simulink model "sampleModel1837"  (R2023a)
settings: Solver=VariableStepAuto  StartTime=0.0  StopTime=10.0  RelTol=1e-3
libraries: simulink x3, hdlsllib x2
settings Model: Creator=user1  LastModifiedBy=user1

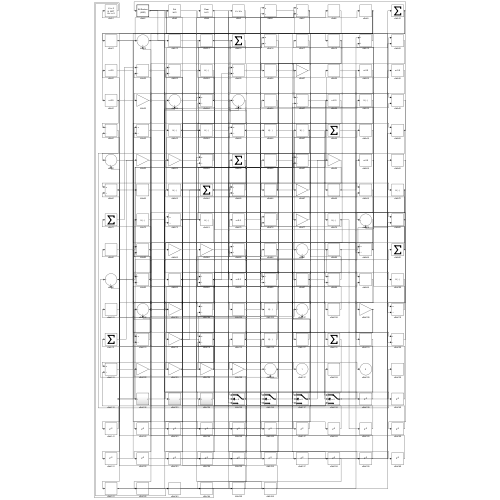
[thumbnail: Simulink's stored preview of the top-level diagram]
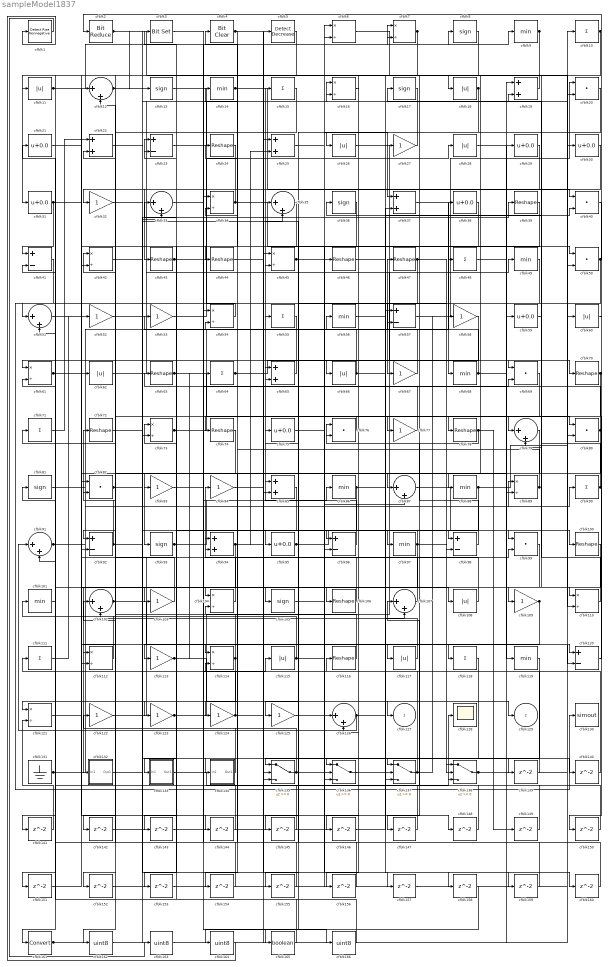
== system sampleModel1837 ==
  cfblk1 : hdlsllib/Logic and Bit Operations/Detect Rise Nonnegative  vinit=0  OutDataTypeStr=boolean
  cfblk{10,15,48,55,64,71,90,111,118} (9 alike) : Sum  Inputs=+
  cfblk{24,39,43..44,46..47,63,70,72,74,78,100,106,116} (14 alike) : Reshape
  cfblk{9,14,49,56,68,86,88,97,101,119} (10 alike) : MinMax
  cfblk{12,33,35,51,79,87,91,102,107,126} (10 alike) : Sum  Inputs=|++
  cfblk{27,32,52..53,58,67,77,83..84,103,109,113,122..125} (16 alike) : Gain
  cfblk{6..7,16,34,42,45,54,61,73,89,104,110,112,114,121} (15 alike) : Product  Inputs=*/  RndMeth=Zero  SaturateOnIntegerOverflow=on
  cfblk{8,13,17,36,81,93,105} (7 alike) : Signum
  cfblk{11,18,26,28,60,62,66,108,115,117} (10 alike) : Abs  SaturateOnIntegerOverflow=off
  cfblk{23,41,57,92,96,98,120} (7 alike) : Sum  Inputs=+-
  cfblk128 : Scope
  cfblk130 : ToWorkspace  VariableName=simout  SaveFormat=Timeseries  SampleTime=-1
  cfblk131 : Ground
  cfblk132 : Subsystem
      settings: LibrarySourceBlock=|
      | hdlsllib/Ports &
      | Subsystems/Subsystem
  cfblk133 : Subsystem
      settings: LibrarySourceBlock=|
      | hdlsllib/Ports &
      | Subsystems/Subsystem
  cfblk134 : Subsystem
      settings: LibrarySourceBlock=|
      | hdlsllib/Ports &
      | Subsystems/Subsystem
  cfblk{135..138} (4 alike) : Switch  SaturateOnIntegerOverflow=off  InputSameDT=off
  cfblk{139..160} (22 alike) : Delay  SampleTime=1
  cfblk161 : DataTypeConversion  SaturateOnIntegerOverflow=off  RndMeth=Floor
  cfblk{162..164,166} (4 alike) : DataTypeConversion  OutDataTypeStr=uint8  SaturateOnIntegerOverflow=off  RndMeth=Floor
  cfblk165 : DataTypeConversion  OutDataTypeStr=boolean  SaturateOnIntegerOverflow=off  RndMeth=Floor
  cfblk{19,22,25,37,65,85,94} (7 alike) : Sum
  cfblk2 : hdlsllib/Logic and Bit Operations/Bit Reduce  mode=AND
  cfblk{20,40,50,69,76,80,82,99} (8 alike) : DotProduct  OutDataTypeStr=Inherit: Inherit via internal rule
  cfblk{21,29..31,38,59,75,95} (8 alike) : Bias  Bias=0.0  SaturateOnIntegerOverflow=off
  cfblk3 : simulink/Logic and Bit Operations/Bit Set  iBit=0
      settings: LibrarySourceBlock=|
      | hdlsllib/Logic and Bit
      | Operations/Bit Set
  cfblk4 : simulink/Logic and Bit Operations/Bit Clear  iBit=0
      settings: LibrarySourceBlock=|
      | hdlsllib/Logic and Bit
      | Operations/Bit Clear
  cfblk5 : simulink/Logic and Bit Operations/Detect Decrease  vinit=0.0  OutDataTypeStr=boolean
      settings: LibrarySourceBlock=|
      | hdlsllib/Logic and Bit
      | Operations/Detect
      | Decrease
  cfblk127 : Outport  VectorParamsAs1DForOutWhenUnconnected=off
  cfblk129 : Outport  Port=2  VectorParamsAs1DForOutWhenUnconnected=off
  wires:
  cfblk109/1 -> cfblk143/1, cfblk165/1
  cfblk52/1 -> cfblk16/1
  cfblk111/1 -> cfblk52/1
  cfblk137/1 -> cfblk116/1, cfblk58/1
  cfblk53/1 -> cfblk28/1
  cfblk124/1 -> cfblk111/1, cfblk129/1, cfblk61/2
  cfblk133/1(Out1) -> cfblk128/1
  cfblk106/1 -> cfblk84/1
  cfblk126/1 -> cfblk91/1, cfblk40/2
  cfblk27/1 -> cfblk26/1
  cfblk80/1 -> cfblk93/1, cfblk63/1
  cfblk102/1 -> cfblk104/1, cfblk135/3
  cfblk71/1 -> cfblk22/1
  cfblk41/1 -> cfblk130/1
  cfblk26/1 -> cfblk70/1
  cfblk131/1 -> cfblk47/1, cfblk99/2
  cfblk120/1 -> cfblk78/1
  cfblk123/1 -> cfblk49/1, cfblk115/1
  cfblk116/1 -> cfblk73/1
  cfblk24/1 -> cfblk43/1
  cfblk100/1 -> cfblk132/1(In1)
  cfblk78/1 -> cfblk76/2, cfblk149/1
  cfblk14/1 -> cfblk40/1, cfblk9/1
  cfblk79/1 -> cfblk114/1
  cfblk20/1 -> cfblk66/1
  cfblk112/1 -> cfblk81/1
  cfblk10/1 -> cfblk109/1, cfblk92/1
  cfblk66/1 -> cfblk23/1, cfblk34/2, cfblk89/2
  cfblk114/1 -> cfblk71/1, cfblk141/1
  cfblk6/1 -> cfblk18/1
  cfblk18/1 -> cfblk37/1, cfblk96/1
  cfblk86/1 -> cfblk118/1, cfblk154/1
  cfblk2/1 -> cfblk13/1, cfblk107/2, cfblk110/2, cfblk157/1
  cfblk89/1 -> cfblk83/1, cfblk24/1
  cfblk31/1 -> cfblk41/1, cfblk103/1
  cfblk46/1 -> cfblk98/1
  cfblk85/1 -> cfblk124/1
  cfblk64/1 -> cfblk69/1, cfblk57/2
  cfblk4/1 -> cfblk106/1, cfblk44/1
  cfblk138/1 -> cfblk19/1, cfblk80/2
  cfblk5/1 -> cfblk161/1
  cfblk37/1 -> cfblk68/1
  cfblk11/1 -> cfblk8/1, cfblk148/1
  cfblk29/1 -> cfblk117/1
  cfblk113/1 -> cfblk127/1, cfblk64/1
  cfblk96/1 -> cfblk15/1
  cfblk28/1 -> cfblk80/1
  cfblk42/1 -> cfblk97/1
  cfblk13/1 -> cfblk67/1
  cfblk115/1 -> cfblk101/1, cfblk159/1
  cfblk87/1 -> cfblk100/1
  cfblk16/1 -> cfblk136/1
  cfblk55/1 -> cfblk133/1(In1)
  cfblk83/1 -> cfblk34/1
  cfblk50/1 -> cfblk2/1, cfblk96/2
  cfblk57/1 -> cfblk20/1
  cfblk36/1 -> cfblk136/2
  cfblk93/1 -> cfblk85/1, cfblk86/1
  cfblk7/1 -> cfblk31/1, cfblk146/1
  cfblk70/1 -> cfblk79/1, cfblk137/2
  cfblk67/1 -> cfblk33/1
  cfblk62/1 -> cfblk38/1
  cfblk15/1 -> cfblk112/1
  cfblk122/1 -> cfblk45/1
  cfblk77/1 -> cfblk65/1
  cfblk105/1 -> cfblk108/1
  cfblk81/1 -> cfblk56/1
  cfblk19/1 -> cfblk11/1
  cfblk34/1 -> cfblk50/1, cfblk32/1
  cfblk45/1 -> cfblk125/1, cfblk87/2
  cfblk22/1 -> cfblk136/3
  cfblk32/1 -> cfblk134/1(In1)
  cfblk134/1(Out1) -> cfblk122/1
  cfblk73/1 -> cfblk46/1, cfblk65/2, cfblk138/2
  cfblk76/1 -> cfblk74/1
  cfblk12/1 -> cfblk105/1, cfblk16/2
  cfblk63/1 -> cfblk48/1, cfblk119/1
  cfblk44/1 -> cfblk25/1
  cfblk98/1 -> cfblk76/1
  cfblk99/1 -> cfblk126/2
  cfblk125/1 -> cfblk7/1
  cfblk43/1 -> cfblk45/2, cfblk138/1
  cfblk54/1 -> cfblk51/1
  cfblk97/1 -> cfblk95/1, cfblk135/2, cfblk139/1
  cfblk92/1 -> cfblk72/1, cfblk90/1
  cfblk103/1 -> cfblk22/2
  cfblk117/1 -> cfblk102/2
  cfblk65/1 -> cfblk61/1
  cfblk35/1 -> cfblk123/1
  cfblk33/1 -> cfblk7/2
  cfblk91/1 -> cfblk12/1, cfblk89/1
  cfblk47/1 -> cfblk98/2, cfblk135/1, cfblk137/3
  cfblk107/1 -> cfblk14/1
  cfblk121/1 -> cfblk82/1
  cfblk51/1 -> cfblk62/1
  cfblk104/1 -> cfblk94/1
  cfblk101/1 -> cfblk21/1
  cfblk88/1 -> cfblk30/1, cfblk153/1
  cfblk95/1 -> cfblk99/1, cfblk55/1
  cfblk94/1 -> cfblk121/1, cfblk69/2, cfblk25/2
  cfblk110/1 -> cfblk19/2
  cfblk48/1 -> cfblk120/1
  cfblk9/1 -> cfblk77/1, cfblk88/1, cfblk73/2, cfblk92/2
  cfblk25/1 -> cfblk27/1
  cfblk108/1 -> cfblk75/1
  cfblk132/1(Out1) -> cfblk39/1
  cfblk90/1 -> cfblk36/1, cfblk17/1
  cfblk58/1 -> cfblk85/2
  cfblk38/1 -> cfblk113/1
  cfblk40/1 -> cfblk110/1
  cfblk39/1 -> cfblk112/2
  cfblk135/1 -> cfblk53/1, cfblk138/3
  cfblk49/1 -> cfblk137/1
  cfblk21/1 -> cfblk87/1
  cfblk59/1 -> cfblk79/2
  cfblk68/1 -> cfblk59/1, cfblk54/2
  cfblk61/1 -> cfblk120/2, cfblk151/1
  cfblk82/1 -> cfblk42/1, cfblk35/2
  cfblk75/1 -> cfblk6/1
  cfblk23/1 -> cfblk10/1
  cfblk139/1 -> cfblk102/1
  cfblk136/1 -> cfblk140/1
  cfblk140/1 -> cfblk114/2
  cfblk141/1 -> cfblk121/2
  cfblk69/1 -> cfblk142/1
  cfblk142/1 -> cfblk37/2
  cfblk143/1 -> cfblk126/1
  cfblk72/1 -> cfblk144/1
  cfblk144/1 -> cfblk23/2
  cfblk17/1 -> cfblk145/1
  cfblk145/1 -> cfblk51/2
  cfblk146/1 -> cfblk57/1
  cfblk8/1 -> cfblk147/1
  cfblk147/1 -> cfblk94/2
  cfblk148/1 -> cfblk107/1
  cfblk149/1 -> cfblk104/2
  cfblk60/1 -> cfblk150/1
  cfblk150/1 -> cfblk12/2
  cfblk151/1 -> cfblk42/2
  cfblk30/1 -> cfblk152/1
  cfblk152/1 -> cfblk20/2
  cfblk153/1 -> cfblk6/2
  cfblk154/1 -> cfblk54/1
  cfblk118/1 -> cfblk155/1
  cfblk155/1 -> cfblk82/2
  cfblk119/1 -> cfblk156/1
  cfblk156/1 -> cfblk91/2
  cfblk157/1 -> cfblk50/2
  cfblk56/1 -> cfblk158/1
  cfblk159/1 -> cfblk35/1
  cfblk84/1 -> cfblk160/1
  cfblk160/1 -> cfblk4/1
  cfblk161/1 -> cfblk33/2, cfblk60/1
  cfblk74/1 -> cfblk162/1
  cfblk162/1 -> cfblk5/1
  cfblk1/1 -> cfblk163/1
  cfblk163/1 -> cfblk29/1
  cfblk158/1 -> cfblk164/1
  cfblk164/1 -> cfblk1/1
  cfblk165/1 -> cfblk3/1
  cfblk3/1 -> cfblk166/1
  cfblk166/1 -> cfblk41/2

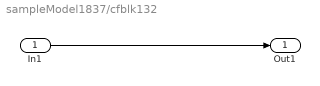
== system sampleModel1837/cfblk132 ==
  In1 : Inport
  Out1 : Outport
  wires:
  In1/1 -> Out1/1

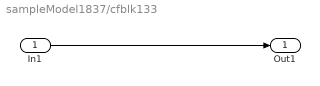
== system sampleModel1837/cfblk133 ==
  In1 : Inport
  Out1 : Outport
  wires:
  In1/1 -> Out1/1

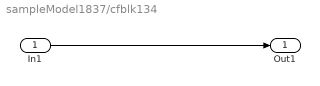
== system sampleModel1837/cfblk134 ==
  In1 : Inport
  Out1 : Outport
  wires:
  In1/1 -> Out1/1
